simulink model "two_tanks_model_PID_saturation_antiwindup_review"  (R2018b)
settings: Solver=FixedStepAuto  StartTime=0.0  StopTime=2400  FixedStep=0.1  RelTol=1e-3
model workspace (MATLAB code in the model file):
  | A1 = 1;
  | a1 = 0.1*0.1;
  | A2 = A1;
  | a2 = a1;
  | h10 = 1;
  | h20=1;
settings Model: PacingRate=100  Creator=kjartan  LastModifiedBy=kjartan

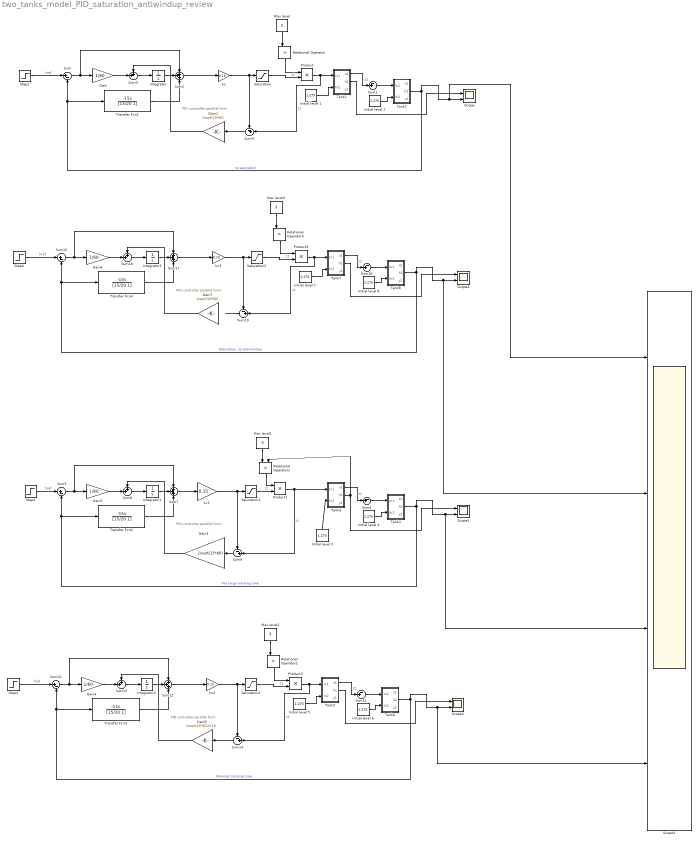
== system two_tanks_model_PID_saturation_antiwindup_review ==
  note: PID controller parallel form
  note: PID controller parallel form
  note: PID controller parallel form
  note: PID controller parallel form
  Gain{,2,4,6} (4 alike) : Gain  Gain=1/60
  Gain1 : Gain  Gain=1/sqrt(15*60)
  Gain3 : Gain  Gain=1/sqrt(15*60)
  Gain5 : Gain  Gain=1/sqrt(15*60)/0.15
  Gain7 : Gain  Gain=1/sqrt(15*60)
  Initial level {1..8} (8 alike) : Constant  Value=1.275
  Integrator{,1..3} (4 alike) : Integrator
  Max level{,1..3} (4 alike) : Constant  Value=3
  Product{,1..3} (4 alike) : Product
  Relational Operator{,1..3} (4 alike) : RelationalOperator  Operator=>  OutDataTypeStr=boolean  RndMeth=Simplest
  Saturation : Saturate  UpperLimit=10  LowerLimit=0
  Saturation1 : Saturate  UpperLimit=0.07  LowerLimit=0
  Saturation2 : Saturate  UpperLimit=0.07  LowerLimit=0
  Saturation3 : Saturate  UpperLimit=0.07  LowerLimit=0
  Scope{,1..2,4} (4 alike) : Scope  NumInputPorts=2
  Scope3 : Scope  NumInputPorts=4
  Step{1..4} (4 alike) : Step  Time=800  Before=1.275  After=2  SampleTime=0
  Sum{,5,10,15} (4 alike) : Sum  Inputs=|+-
  Sum{1,4,6,9,11,14,16,19} (8 alike) : Sum  Inputs=-+|
  Sum{2,7,12,17} (4 alike) : Sum  Inputs=+++
  Sum{3,8,13,18} (4 alike) : Sum  Inputs=++|
  Tank1 : Subsystem
  Tank2 : Subsystem
  Tank3 : Subsystem
  Tank4 : Subsystem
  Tank5 : Subsystem
  Tank6 : Subsystem
  Tank7 : Subsystem
  Tank8 : Subsystem
  Transfer Fcn{1..4} (4 alike) : TransferFcn  Numerator=[-15 0]  Denominator=[15/20 1]
  kc{,1..3} (4 alike) : Gain  Gain=0.15
  wires:
  Tank1/1(x1) -> Sum1/2  "z2"
  Tank1/2(h1) -> Scope/1
  Tank2/2(h2) -> Scope3/1, Scope/2, Sum/2, Transfer Fcn1/1  "no saturation"
  Sum1/1 -> Tank2/1(In1)
  Step1/1 -> Sum/1  "href"
  Sum/1 -> Gain/1, Sum2/1
  Product/1 -> Sum4/2, Tank1/1(In1)  "z1"
  kc/1 -> Saturation/1, Sum4/1
  Initial level 2/1 -> Tank2/2(In2)
  Initial level 1/1 -> Tank1/2(In2)
  Transfer Fcn1/1 -> Sum2/3
  Sum2/1 -> kc/1
  Integrator/1 -> Sum2/2
  Gain/1 -> Sum3/2
  Max level/1 -> Relational Operator/1
  Saturation/1 -> Product/2  "z1"
  Relational Operator/1 -> Product/1
  Sum3/1 -> Integrator/1
  Sum4/1 -> Gain1/1
  Gain1/1 -> Sum3/1
  Initial level 3/1 -> Tank3/2(In2)
  Sum8/1 -> Integrator1/1
  Integrator1/1 -> Sum7/2
  Product1/1 -> Tank3/1(In1), Sum9/2  "z1"
  Saturation1/1 -> Product1/2  "z1"
  Initial level 4/1 -> Tank4/2(In2)
  Gain2/1 -> Sum8/2
  Sum7/1 -> kc1/1
  Step2/1 -> Sum5/1  "href"
  kc1/1 -> Saturation1/1, Sum9/1
  Tank3/1(x1) -> Sum6/2  "z2"
  Transfer Fcn2/1 -> Sum7/3
  Tank4/2(h2) -> Scope3/3, Scope1/2, Sum5/2, Transfer Fcn2/1  "Too large tracking time"
  Sum6/1 -> Tank4/1(In1)
  Sum5/1 -> Gain2/1, Sum7/1
  Max level1/1 -> Relational Operator1/1
  Relational Operator1/1 -> Product1/1
  Gain3/1 -> Sum8/1
  Sum9/1 -> Gain3/1
  Initial level 5/1 -> Tank5/2(In2)
  Sum13/1 -> Integrator2/1
  Integrator2/1 -> Sum12/2
  Product2/1 -> Sum14/2, Tank5/1(In1)  "z1"
  Saturation2/1 -> Product2/2  "z1"
  Initial level 6/1 -> Tank6/2(In2)
  Gain4/1 -> Sum13/2
  Sum12/1 -> kc2/1
  Step3/1 -> Sum10/1  "href"
  kc2/1 -> Saturation2/1, Sum14/1
  Tank5/1(x1) -> Sum11/2  "z2"
  Transfer Fcn3/1 -> Sum12/3
  Tank6/2(h2) -> Scope3/4, Scope2/2, Sum10/2, Transfer Fcn3/1  "Nominal tracking time"
  Sum11/1 -> Tank6/1(In1)
  Sum10/1 -> Gain4/1, Sum12/1
  Max level2/1 -> Relational Operator2/1
  Relational Operator2/1 -> Product2/1
  Gain5/1 -> Sum13/1
  Tank5/2(h1) -> Scope2/1
  Sum14/1 -> Gain5/1
  Product3/1 -> Sum19/2, Tank7/1(In1)  "z1"
  Saturation3/1 -> Product3/2  "z1"
  Initial level 7/1 -> Tank7/2(In2)
  Sum18/1 -> Integrator3/1
  Initial level 8/1 -> Tank8/2(In2)
  Gain6/1 -> Sum18/2
  Sum17/1 -> kc3/1
  Sum15/1 -> Gain6/1, Sum17/1
  Tank7/1(x1) -> Sum16/2  "z2"
  Step4/1 -> Sum15/1  "href"
  kc3/1 -> Saturation3/1, Sum19/1
  Transfer Fcn4/1 -> Sum17/3
  Tank8/2(h2) -> Scope3/2, Scope4/2, Sum15/2, Transfer Fcn4/1  "Saturation, no anti-windup"
  Sum16/1 -> Tank8/1(In1)
  Integrator3/1 -> Sum17/2
  Max level3/1 -> Relational Operator3/1
  Relational Operator3/1 -> Product3/1
  Gain7/1 -> Sum18/1
  Tank7/2(h1) -> Scope4/1
  Sum19/1 -> ?
  Tank3/2(h1) -> Scope1/1, Relational Operator1/2

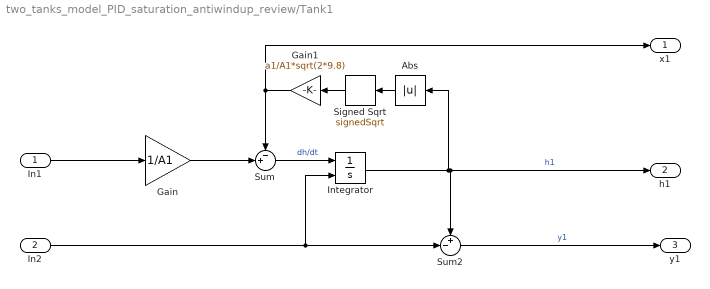
== system two_tanks_model_PID_saturation_antiwindup_review/Tank1 ==
  In1 : Inport
  In2 : Inport  Port=2
  Abs : Abs
  Gain : Gain  Gain=1/A1
  Gain1 : Gain  Gain=a1/A1*sqrt(2*9.8)
  Integrator : Integrator  InitialConditionSource=external  InitialCondition=h10
  Signed Sqrt : Sqrt  Operator=signedSqrt  SaturateOnIntegerOverflow=on
  Sum : Sum  Inputs=-+|
  Sum2 : Sum  Inputs=+-|
  x1 : Outport
  h1 : Outport  Port=2
  y1 : Outport  Port=3
  wires:
  Gain1/1 -> x1/1, Sum/1
  Gain/1 -> Sum/2
  Sum/1 -> Integrator/1  "dh/dt"
  In1/1 -> Gain/1
  Sum2/1 -> y1/1  "y1"
  Signed Sqrt/1 -> Gain1/1
  Integrator/1 -> h1/1, Sum2/1, Abs/1  "h1"
  Abs/1 -> Signed Sqrt/1
  In2/1 -> Sum2/2, Integrator/2

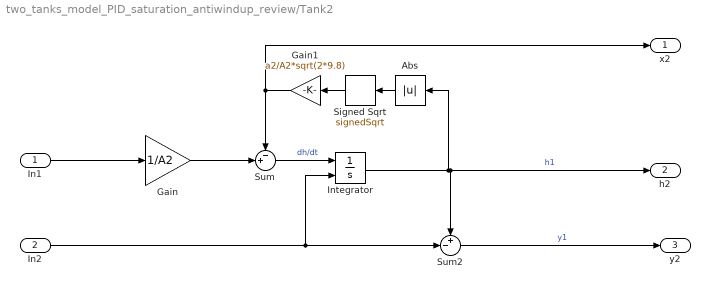
== system two_tanks_model_PID_saturation_antiwindup_review/Tank2 ==
  In1 : Inport
  In2 : Inport  Port=2
  Abs : Abs
  Gain : Gain  Gain=1/A2
  Gain1 : Gain  Gain=a2/A2*sqrt(2*9.8)
  Integrator : Integrator  InitialConditionSource=external  InitialCondition=h10
  Signed Sqrt : Sqrt  Operator=signedSqrt  SaturateOnIntegerOverflow=on
  Sum : Sum  Inputs=-+|
  Sum2 : Sum  Inputs=+-|
  x2 : Outport
  h2 : Outport  Port=2
  y2 : Outport  Port=3
  wires:
  Gain1/1 -> x2/1, Sum/1
  Gain/1 -> Sum/2
  Sum/1 -> Integrator/1  "dh/dt"
  In1/1 -> Gain/1
  Sum2/1 -> y2/1  "y1"
  Signed Sqrt/1 -> Gain1/1
  Integrator/1 -> h2/1, Sum2/1, Abs/1  "h1"
  Abs/1 -> Signed Sqrt/1
  In2/1 -> Sum2/2, Integrator/2

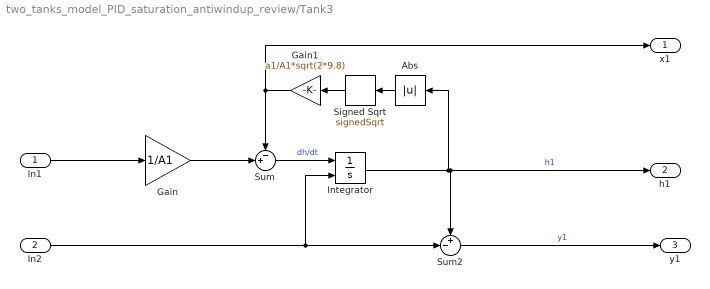
== system two_tanks_model_PID_saturation_antiwindup_review/Tank3 ==
  In1 : Inport
  In2 : Inport  Port=2
  Abs : Abs
  Gain : Gain  Gain=1/A1
  Gain1 : Gain  Gain=a1/A1*sqrt(2*9.8)
  Integrator : Integrator  InitialConditionSource=external  InitialCondition=h10
  Signed Sqrt : Sqrt  Operator=signedSqrt  SaturateOnIntegerOverflow=on
  Sum : Sum  Inputs=-+|
  Sum2 : Sum  Inputs=+-|
  x1 : Outport
  h1 : Outport  Port=2
  y1 : Outport  Port=3
  wires:
  Gain1/1 -> x1/1, Sum/1
  Gain/1 -> Sum/2
  Sum/1 -> Integrator/1  "dh/dt"
  In1/1 -> Gain/1
  Sum2/1 -> y1/1  "y1"
  Signed Sqrt/1 -> Gain1/1
  Integrator/1 -> h1/1, Sum2/1, Abs/1  "h1"
  Abs/1 -> Signed Sqrt/1
  In2/1 -> Sum2/2, Integrator/2

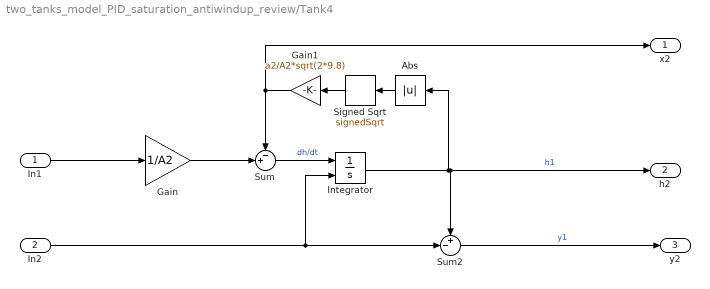
== system two_tanks_model_PID_saturation_antiwindup_review/Tank4 ==
  In1 : Inport
  In2 : Inport  Port=2
  Abs : Abs
  Gain : Gain  Gain=1/A2
  Gain1 : Gain  Gain=a2/A2*sqrt(2*9.8)
  Integrator : Integrator  InitialConditionSource=external  InitialCondition=h10
  Signed Sqrt : Sqrt  Operator=signedSqrt  SaturateOnIntegerOverflow=on
  Sum : Sum  Inputs=-+|
  Sum2 : Sum  Inputs=+-|
  x2 : Outport
  h2 : Outport  Port=2
  y2 : Outport  Port=3
  wires:
  Gain1/1 -> x2/1, Sum/1
  Gain/1 -> Sum/2
  Sum/1 -> Integrator/1  "dh/dt"
  In1/1 -> Gain/1
  Sum2/1 -> y2/1  "y1"
  Signed Sqrt/1 -> Gain1/1
  Integrator/1 -> h2/1, Sum2/1, Abs/1  "h1"
  Abs/1 -> Signed Sqrt/1
  In2/1 -> Sum2/2, Integrator/2

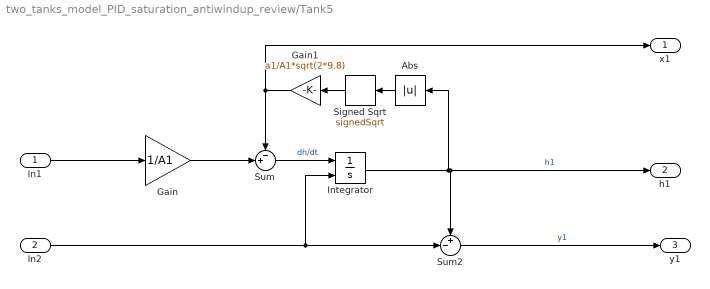
== system two_tanks_model_PID_saturation_antiwindup_review/Tank5 ==
  In1 : Inport
  In2 : Inport  Port=2
  Abs : Abs
  Gain : Gain  Gain=1/A1
  Gain1 : Gain  Gain=a1/A1*sqrt(2*9.8)
  Integrator : Integrator  InitialConditionSource=external  InitialCondition=h10
  Signed Sqrt : Sqrt  Operator=signedSqrt  SaturateOnIntegerOverflow=on
  Sum : Sum  Inputs=-+|
  Sum2 : Sum  Inputs=+-|
  x1 : Outport
  h1 : Outport  Port=2
  y1 : Outport  Port=3
  wires:
  Gain1/1 -> x1/1, Sum/1
  Gain/1 -> Sum/2
  Sum/1 -> Integrator/1  "dh/dt"
  In1/1 -> Gain/1
  Sum2/1 -> y1/1  "y1"
  Signed Sqrt/1 -> Gain1/1
  Integrator/1 -> h1/1, Sum2/1, Abs/1  "h1"
  Abs/1 -> Signed Sqrt/1
  In2/1 -> Sum2/2, Integrator/2

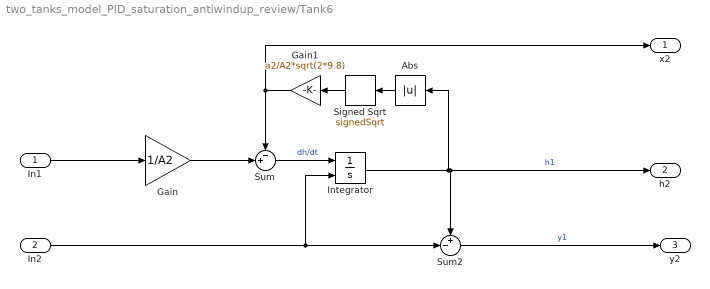
== system two_tanks_model_PID_saturation_antiwindup_review/Tank6 ==
  In1 : Inport
  In2 : Inport  Port=2
  Abs : Abs
  Gain : Gain  Gain=1/A2
  Gain1 : Gain  Gain=a2/A2*sqrt(2*9.8)
  Integrator : Integrator  InitialConditionSource=external  InitialCondition=h10
  Signed Sqrt : Sqrt  Operator=signedSqrt  SaturateOnIntegerOverflow=on
  Sum : Sum  Inputs=-+|
  Sum2 : Sum  Inputs=+-|
  x2 : Outport
  h2 : Outport  Port=2
  y2 : Outport  Port=3
  wires:
  Gain1/1 -> x2/1, Sum/1
  Gain/1 -> Sum/2
  Sum/1 -> Integrator/1  "dh/dt"
  In1/1 -> Gain/1
  Sum2/1 -> y2/1  "y1"
  Signed Sqrt/1 -> Gain1/1
  Integrator/1 -> h2/1, Sum2/1, Abs/1  "h1"
  Abs/1 -> Signed Sqrt/1
  In2/1 -> Sum2/2, Integrator/2

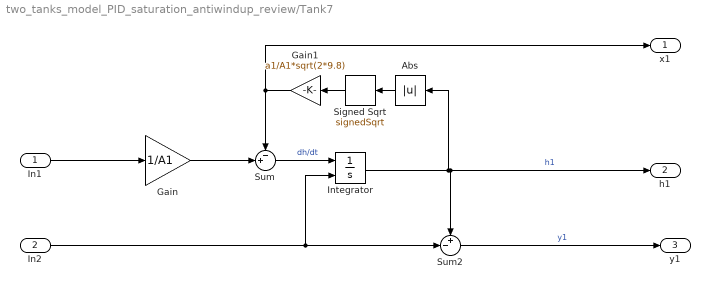
== system two_tanks_model_PID_saturation_antiwindup_review/Tank7 ==
  In1 : Inport
  In2 : Inport  Port=2
  Abs : Abs
  Gain : Gain  Gain=1/A1
  Gain1 : Gain  Gain=a1/A1*sqrt(2*9.8)
  Integrator : Integrator  InitialConditionSource=external  InitialCondition=h10
  Signed Sqrt : Sqrt  Operator=signedSqrt  SaturateOnIntegerOverflow=on
  Sum : Sum  Inputs=-+|
  Sum2 : Sum  Inputs=+-|
  x1 : Outport
  h1 : Outport  Port=2
  y1 : Outport  Port=3
  wires:
  Gain1/1 -> x1/1, Sum/1
  Gain/1 -> Sum/2
  Sum/1 -> Integrator/1  "dh/dt"
  In1/1 -> Gain/1
  Sum2/1 -> y1/1  "y1"
  Signed Sqrt/1 -> Gain1/1
  Integrator/1 -> h1/1, Sum2/1, Abs/1  "h1"
  Abs/1 -> Signed Sqrt/1
  In2/1 -> Sum2/2, Integrator/2

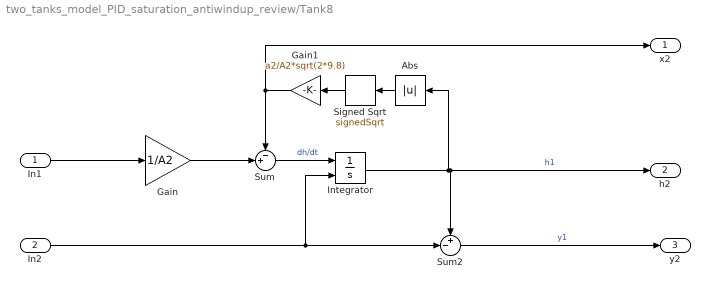
== system two_tanks_model_PID_saturation_antiwindup_review/Tank8 ==
  In1 : Inport
  In2 : Inport  Port=2
  Abs : Abs
  Gain : Gain  Gain=1/A2
  Gain1 : Gain  Gain=a2/A2*sqrt(2*9.8)
  Integrator : Integrator  InitialConditionSource=external  InitialCondition=h10
  Signed Sqrt : Sqrt  Operator=signedSqrt  SaturateOnIntegerOverflow=on
  Sum : Sum  Inputs=-+|
  Sum2 : Sum  Inputs=+-|
  x2 : Outport
  h2 : Outport  Port=2
  y2 : Outport  Port=3
  wires:
  Gain1/1 -> x2/1, Sum/1
  Gain/1 -> Sum/2
  Sum/1 -> Integrator/1  "dh/dt"
  In1/1 -> Gain/1
  Sum2/1 -> y2/1  "y1"
  Signed Sqrt/1 -> Gain1/1
  Integrator/1 -> h2/1, Sum2/1, Abs/1  "h1"
  Abs/1 -> Signed Sqrt/1
  In2/1 -> Sum2/2, Integrator/2
